simulink model "Task1_sim"  (R2024b)
settings: Solver=VariableStepAuto  StartTime=0.0  StopTime=100  RelTol=1e-3
values from neighbouring files (symbols this model uses):
  I = diag([Ix, Iy, Iz])    [Task1.m]    (also in Task2.m; Task3.m; Task4.m)
  w_0 = [0.45, 0.52, 0.52]'    [Task1.m]    (also in Task2.m = [wx_0, wy_0, wz_0]'; Task3.m = [0.1, 0.1, 2]'; Task4.m = [1e-6, 1e-6, 0.02]')
libraries: matrix_library x1
settings Model: Creator=alejandromunozvazquez  LastModifiedBy=alejandromunozvazquez

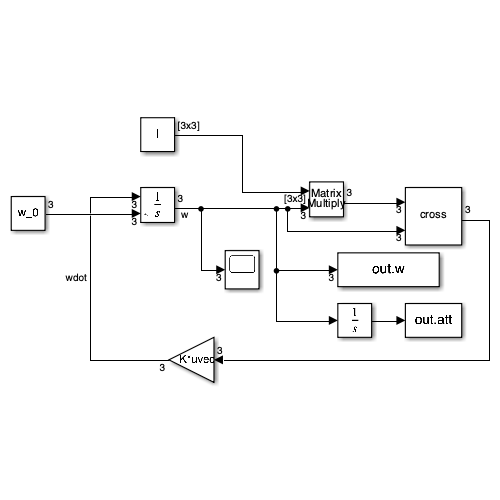
[thumbnail: Simulink's stored preview of the top-level diagram]
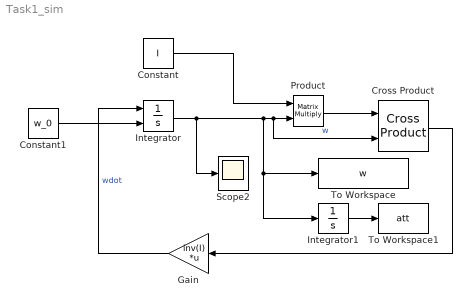
== system Task1_sim ==
  Constant : Constant  Value=I
  Constant1 : Constant  Value=w_0
  Cross Product : matrix_library/Cross Product
  Gain : Gain  Gain=inv(I)  Multiplication=Matrix(K*u) (u vector)
  Integrator : Integrator  InitialConditionSource=external
  Integrator1 : Integrator
  Product : Product  Multiplication=Matrix(*)
  Scope2 : Scope
  To Workspace : ToWorkspace  VariableName=w  SampleTime=-1
  To Workspace1 : ToWorkspace  VariableName=att  SampleTime=-1
  wires:
  Gain/1 -> Integrator/1  "wdot"
  Integrator/1 -> Scope2/1, Product/2, Cross Product/2, Integrator1/1, To Workspace/1  "w"
  Constant/1 -> Product/1
  Product/1 -> Cross Product/1
  Cross Product/1 -> Gain/1
  Constant1/1 -> Integrator/2
  Integrator1/1 -> To Workspace1/1
